simulink model "kontrollflussdiagramm"  (R2015b)
settings: Solver=VariableStepAuto  StartTime=0.0  StopTime=inf  RelTol=1e-3
settings Model: Creator=scco1019  LastModifiedBy=scco1019

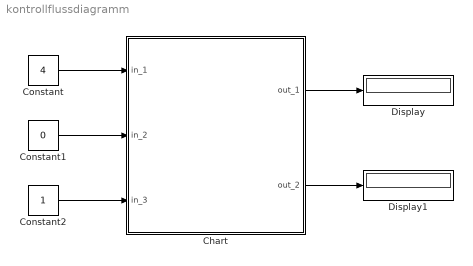
== system kontrollflussdiagramm ==
  Chart : Stateflow chart  TreatAsAtomicUnit=on
  Constant : Constant  Value=4
  Constant1 : Constant  Value=0
  Constant2 : Constant
  Display : Display
  Display1 : Display
  wires:
  Constant/1 -> Chart/1(in_1)
  Constant1/1 -> Chart/2(in_2)
  Constant2/1 -> Chart/3(in_3)
  Chart/1(out_1) -> Display/1
  Chart/2(out_2) -> Display1/1

== stateflow chart kontrollflussdiagramm/Chart ==
  (default) -> (junction 9)
  (junction 9) -> (junction 18) [order 2] : {out_1=0; out_2=0;}
  (junction 9) -> (junction 20) [order 1] : [in_1 || in_2]
  (junction 18) -> (junction 22)
  (junction 20) -> (junction 22) [order 2] : {out_1=1; out_2=1;}
  (junction 20) -> (junction 24) [order 1] : [in_1==4]
  (junction 22) -> (junction 27)
  (junction 24) -> (junction 27) : {out_1=3; out_2=1;}
  data: in_1 input; in_2 input; in_3 input; out_1 output; out_2 output
